simulink model "FTC_PID_VuForiaController"  (R2015b)
settings: Solver=VariableStepAuto  StartTime=0.0  StopTime=1000  FixedStep=10  RelTol=1e-3
libraries: simulink x1
settings Model: Creator=Ryley  LastModifiedBy=Ryley

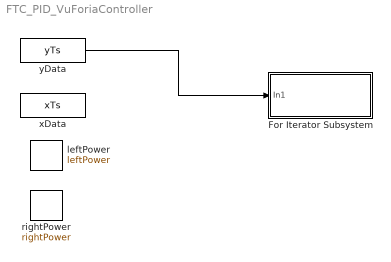
== system FTC_PID_VuForiaController ==
  For Iterator Subsystem : Subsystem  TreatAsAtomicUnit=on
  "leftPower " : DataStoreMemory  DataStoreName=leftPower  ReadBeforeWriteMsg=warning  WriteAfterWriteMsg=warning  WriteAfterReadMsg=warning  InitialValue=0.5
  "rightPower " : DataStoreMemory  DataStoreName=rightPower  ReadBeforeWriteMsg=warning  WriteAfterWriteMsg=warning  WriteAfterReadMsg=warning  InitialValue=0.5
  "xData " : FromWorkspace  VariableName=xTs  SampleTime=0
  yData : FromWorkspace  VariableName=yTs  SampleTime=0
  wires:
  yData/1 -> For Iterator Subsystem/1(In1)

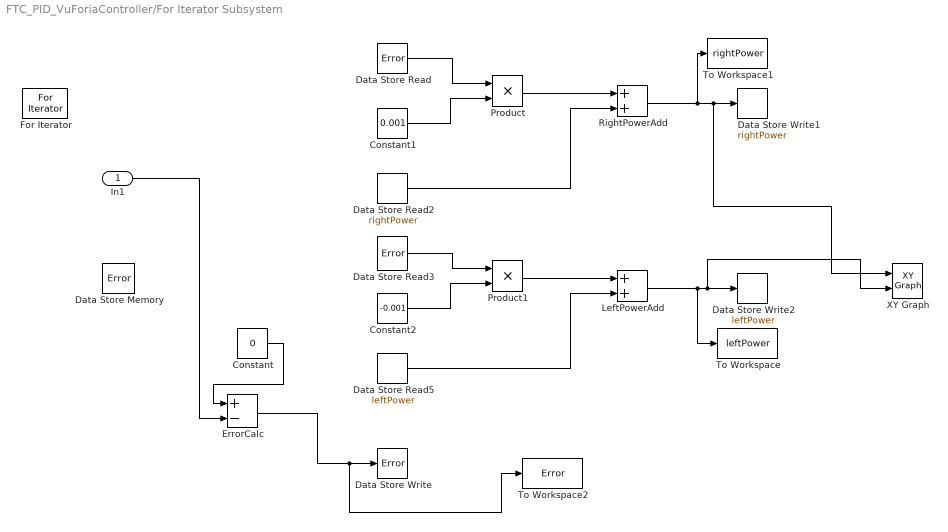
== system FTC_PID_VuForiaController/For Iterator Subsystem ==
  In1 : Inport
  Constant : Constant  Value=0
  Constant1 : Constant  Value=0.001
  Constant2 : Constant  Value=-0.001
  Data Store Memory : DataStoreMemory  DataStoreName=Error  ReadBeforeWriteMsg=warning  WriteAfterWriteMsg=warning  WriteAfterReadMsg=warning
  Data Store Read : DataStoreRead  DataStoreName=Error
  Data Store Read2 : DataStoreRead  DataStoreName=rightPower
  Data Store Read3 : DataStoreRead  DataStoreName=Error
  Data Store Read5 : DataStoreRead  DataStoreName=leftPower
  Data Store Write : DataStoreWrite  DataStoreName=Error
  Data Store Write1 : DataStoreWrite  DataStoreName=rightPower
  Data Store Write2 : DataStoreWrite  DataStoreName=leftPower
  ErrorCalc : Sum  Inputs=+-
  For Iterator : ForIterator  IterationLimit=1000
  "LeftPowerAdd " : Sum
  Product : Product
  Product1 : Product
  "RightPowerAdd " : Sum
  To Workspace : ToWorkspace  VariableName=leftPower  SaveFormat=Timeseries  SampleTime=-1
  To Workspace1 : ToWorkspace  VariableName=rightPower  SaveFormat=Timeseries  SampleTime=-1
  To Workspace2 : ToWorkspace  VariableName=Error  SaveFormat=Timeseries  SampleTime=-1
  XY Graph : simulink/Sinks/XY Graph  xmin=-10  xmax=10  ymin=-10  ymax=10  st=-1
  wires:
  In1/1 -> ErrorCalc/2
  Constant/1 -> ErrorCalc/1
  ErrorCalc/1 -> To Workspace2/1, Data Store Write/1
  Data Store Read/1 -> Product/1
  Constant1/1 -> Product/2
  Product/1 -> "RightPowerAdd "/1
  Data Store Read2/1 -> "RightPowerAdd "/2
  "RightPowerAdd "/1 -> To Workspace1/1, XY Graph/1, Data Store Write1/1
  Data Store Read3/1 -> Product1/1
  Constant2/1 -> Product1/2
  Product1/1 -> "LeftPowerAdd "/1
  Data Store Read5/1 -> "LeftPowerAdd "/2
  "LeftPowerAdd "/1 -> To Workspace/1, XY Graph/2, Data Store Write2/1
